simulink subsystem "HIL_Send_TCP_Data_2021a"  (R2021b)
settings: Solver=VariableStepAuto  StartTime=0.0  StopTime=10.0  RelTol=1e-3
model mask{mi_ip=mi_ip, mi_port=mi_port, f=0}
  mask prompts: mi_ip "Server IP"; mi_port "Server Port"; f "Sampling Frequency"
libraries: etargetslib x2, slrealtimeiplib x1
settings Model: Creator=ramuj  LastModifiedBy=Hyperloop UPV
settings DebuggingCC: UnconnectedInputMsg=none  UnconnectedOutputMsg=none  UnconnectedLineMsg=none
settings ModelReferenceCC: EnableRefExpFcnMdlSchedulingChecks=off
settings RTWCC: DLArmComputeVersion=20.02.1

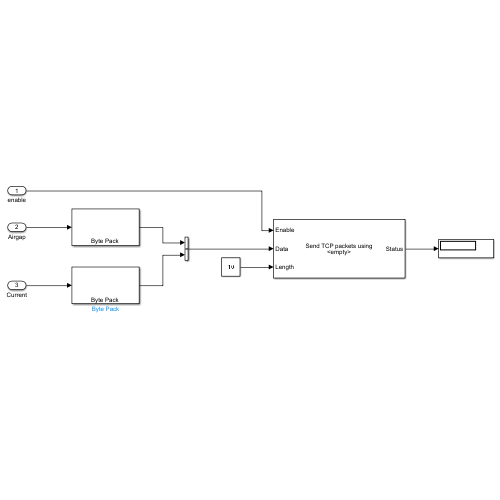
[thumbnail: Simulink's stored preview of the top-level diagram]
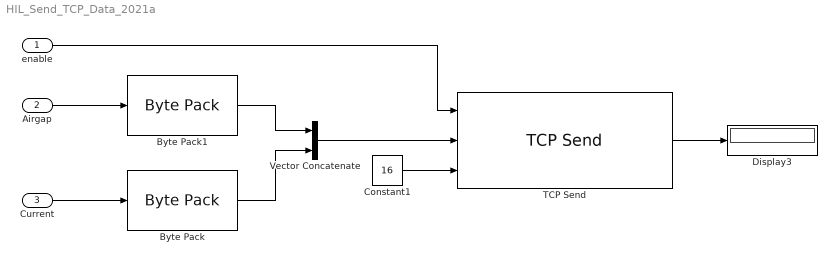
== system HIL_Send_TCP_Data_2021a ==
  enable : Inport  OutDataTypeStr=double
  Airgap : Inport  Port=2
  Current : Inport  Port=3
  Byte Pack : etargetslib/Byte Pack  datatypes={'double'}  byteAlign=1
  Byte Pack1 : etargetslib/Byte Pack  datatypes={'double'}  byteAlign=1
  Constant1 : Constant  Value=16
  Display3 : Display
  TCP Send : slrealtimeiplib/TCP Send  socketAddPortVal=<empty>  sampleTime=1/f
      settings: SourceProductBaseCode=XP
  Vector Concatenate : Concatenate
  wires:
  Airgap/1 -> Byte Pack1/1
  TCP Send/1 -> Display3/1
  enable/1 -> TCP Send/1
  Current/1 -> Byte Pack/1
  Constant1/1 -> TCP Send/3
  Vector Concatenate/1 -> TCP Send/2
  Byte Pack1/1 -> Vector Concatenate/1
  Byte Pack/1 -> Vector Concatenate/2
